simulink model "P_I"  (R2022a)
settings: Solver=VariableStepAuto  StartTime=0.0  StopTime=30  RelTol=1e-3
settings Model: Creator=anthony  LastModifiedBy=anthony

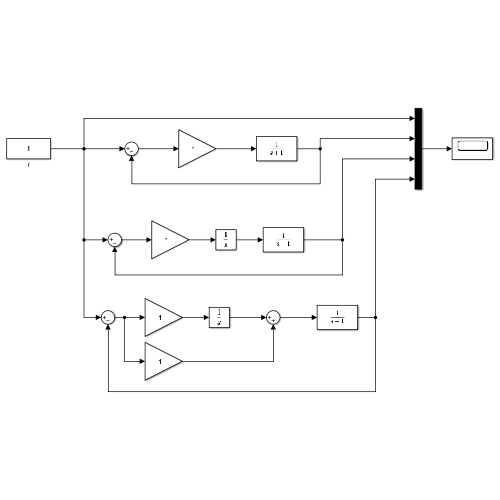
[thumbnail: Simulink's stored preview of the top-level diagram]
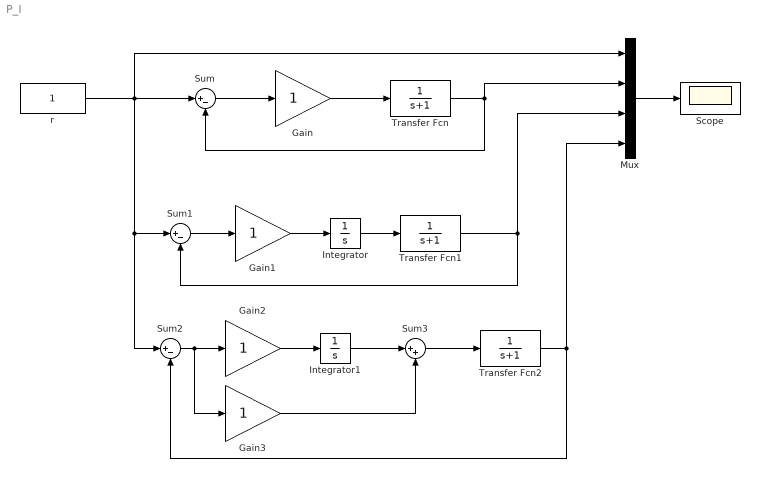
== system P_I ==
  Gain{,1..3} (4 alike) : Gain
  Integrator : Integrator
  Integrator1 : Integrator
  Mux : Mux
  Scope : Scope
  Sum : Sum  Inputs=|+-
  Sum1 : Sum  Inputs=|+-
  Sum2 : Sum  Inputs=|+-
  Sum3 : Sum  Inputs=|++
  Transfer Fcn : TransferFcn  Denominator=[1 1]
  Transfer Fcn1 : TransferFcn  Denominator=[1 1]
  Transfer Fcn2 : TransferFcn  Denominator=[1 1]
  r : Constant
  wires:
  Mux/1 -> Scope/1
  Sum/1 -> Gain/1
  Gain/1 -> Transfer Fcn/1
  Transfer Fcn/1 -> Mux/2, Sum/2
  Transfer Fcn1/1 -> Sum1/2, Mux/3
  Sum1/1 -> Gain1/1
  r/1 -> Sum2/1, Sum1/1, Mux/1, Sum/1
  Gain1/1 -> Integrator/1
  Integrator/1 -> Transfer Fcn1/1
  Gain2/1 -> Integrator1/1
  Sum2/1 -> Gain3/1, Gain2/1
  Transfer Fcn2/1 -> Mux/4, Sum2/2
  Gain3/1 -> Sum3/2
  Integrator1/1 -> Sum3/1
  Sum3/1 -> Transfer Fcn2/1
